simulink model "closedLoopR2019"  (Simulink 10.0)
settings: Solver=FixedStepAuto  StartTime=0.0  StopTime=inf  FixedStep=0.001  RelTol=1e-3
settings Model: Creator=marko  LastModifiedBy=Marko
settings DataIOCC: SaveFormat=Dataset  ReturnWorkspaceOutputs=on
settings OptimizationCC: LifeSpan=auto
settings DebuggingCC: UnderspecifiedInitializationDetection=Simplified  MergeDetectMultiDrivingBlocksExec=error  SFUnexpectedBacktrackingDiag=error  SFNoUnconditionalDefaultTransitionDiag=error  SFExecutionAtInitializationDiag=warning  ArithmeticOperatorsInVariantConditions=error
settings HardwareCC: ProdBitPerPointer=64  ProdBitPerSizeT=64  ProdBitPerPtrDiffT=64  ProdLargestAtomicFloat=Float  ProdIntDivRoundTo=Zero  ProdEndianess=LittleEndian  ProdWordSize=64  ProdHWDeviceType=Intel->x86-64 (Windows64)
settings ModelReferenceCC: PropagateSignalLabelsOutOfModel=on
settings SFSimCC: SimUseLocalCustomCode=on  CustomCodeUndefinedFunction=FilterOut
settings RTWCC: RTWUseLocalCustomCode=on
settings CodeAppCC: StateflowObjectComments=off
settings GRTTargetCC: TargetLangStandard=C99 (ISO)  CombineOutputUpdateFcns=on  GRTInterface=off
settings ConfigComp: CovMetricSettings=dwe  CovSaveCumulativeToWorkspaceVar=off  CovSaveSingleToWorkspaceVar=off

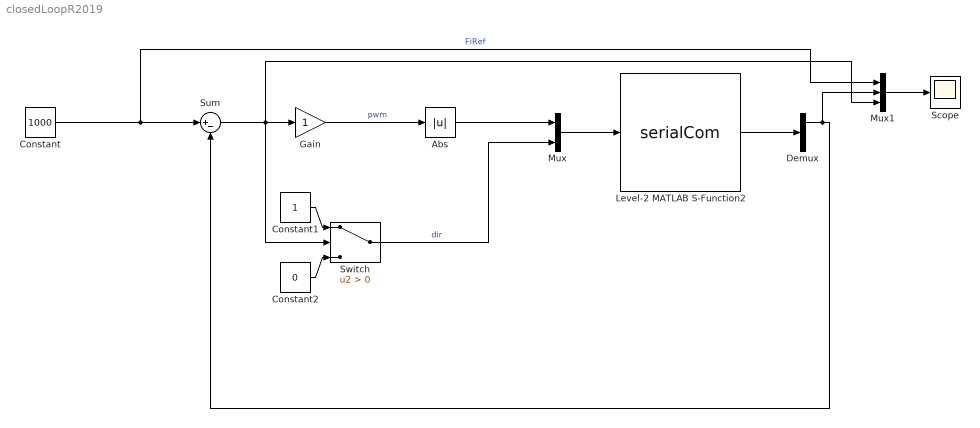
== system closedLoopR2019 ==
  Abs : Abs
  Constant : Constant  Value=1000
  Constant1 : Constant
  Constant2 : Constant  Value=0
  Demux : Demux  Outputs=2
  Gain : Gain
  Level-2 MATLAB S-Function2 : M-S-Function  FunctionName=serialCom  Parameters='COM9', 115200
      mask Display: image('FlexDrive1.png'); % Use "Edit Image" on toolstrip to change.
  Mux : Mux  Inputs=2
  Mux1 : Mux  Inputs=3
  Scope : Scope
  Sum : Sum  Inputs=|+-
  Switch : Switch  Criteria=u2 > Threshold
  wires:
  Level-2 MATLAB S-Function2/1 -> Demux/1
  Mux/1 -> Level-2 MATLAB S-Function2/1
  Constant/1 -> Mux1/1, Sum/1  "FiRef"
  Sum/1 -> Mux1/3, Switch/2, Gain/1
  Demux/1 -> Mux1/2, Sum/2
  Gain/1 -> Abs/1  "pwm"
  Switch/1 -> Mux/2  "dir"
  Constant1/1 -> Switch/1
  Constant2/1 -> Switch/3
  Mux1/1 -> Scope/1
  Abs/1 -> Mux/1
